simulink model "Model_kalmanTest"  (R2014b)
settings: Solver=ode3  StartTime=0.0  StopTime=T_max  FixedStep=h  RelTol=1e-3
values from neighbouring files (symbols this model uses):
  b = 0.1    [Input_LQR.m]    (also in TestKalman.m; TestSuper.m; TestVahidComparison.m; parameter.m)
  delta = cell(1,length(L_sup))    [TestSuper.m]
  g = 9.81    [Input_LQR.m]    (also in TestKalman.m; TestSuper.m; TestVahidComparison.m; parameter.m = 9.8)
  gamma = cell(1,length(L_sup))    [TestSuper.m]
  h = 0.01    [Input_LQR.m]    (also in TestKalman.m = 0.001; TestSuper.m = 0.001; TestVahidComparison.m = 0.001; parameter.m)
  H = [1 0 0 0 0 0 ... (first row only)    [Input_LQR.m]    (also in TestKalman.m; TestSuper.m; TestVahidComparison.m)
  K = lqr(A, B, Q, R)    [Input_LQR.m]    (also in TestKalman.m; TestSuper.m)
  k = 0.15    [Input_LQR.m]    (also in TestKalman.m; TestSuper.m; TestVahidComparison.m; parameter.m)
  L = 1.4    [Input_LQR.m]    (also in TestKalman.m; TestSuper.m = 1.025; TestVahidComparison.m)
  M = 1    [Input_LQR.m]    (also in TestKalman.m; TestSuper.m; TestVahidComparison.m; parameter.m)
  m = 3/4    (= 0.75)    [Input_LQR.m]    (also in TestKalman.m; TestSuper.m; TestVahidComparison.m; parameter.m)
  P_0 = diag([1,1,1,1,1,1])*0.00001    [Input_LQR.m]    (also in TestKalman.m = diag([1,1,1,1,100,100])*0.001; TestSuper.m = diag([1,1,1,1,100,100])*0.001)
  phi = cell(1,length(L_sup))    [TestSuper.m]
  Q_kalman = diag([(0), (0)])    [Input_LQR.m]    (also in TestKalman.m = diag([(10), (10e-4)]); TestSuper.m = diag([(10), (10e-4)]))
  R_kalman = diag([(10e-7), (10e-6)])    [Input_LQR.m]    (also in TestKalman.m = diag([(10e-7), (10e-7)]); TestSuper.m = diag([(10e-7), (10e-7)]))
  theta_0 = 0    [Input_LQR.m]    (also in TestKalman.m = 0.1; TestSuper.m = 0.1; TestVahidComparison.m = 0.1)
  theta_dot0 = 0    [Input_LQR.m]    (also in TestKalman.m; TestSuper.m; TestVahidComparison.m)
  X_0 = [0 0 0 0 0 0]'    [Input_LQR.m]    (also in TestKalman.m = [x_0 theta_0 x_dot0 theta_dot0 0 0]'; TestSuper.m = [x_0 theta_0 x_dot0 theta_dot0 0 0]')
  x_0 = 0    [Input_LQR.m]    (also in TestKalman.m; TestSuper.m; TestVahidComparison.m)
  x_dot0 = 0    [Input_LQR.m]    (also in TestKalman.m; TestSuper.m; TestVahidComparison.m)
  y_0 = [0 0]    [Input_LQR.m]    (also in TestKalman.m; TestSuper.m)
libraries: simulink x6
settings Model: Creator=Erik  LastModifiedBy=Erik
settings SolverCC: AlgebraicLoopSolver=LineSearch
settings OptimizationCC: UseDivisionForNetSlopeComputation=off  SimCompilerOptimization=off
settings DebuggingCC: FrameProcessingCompatibilityMsg=error
settings RTWCC: RTWCompilerOptimization=off
settings ConfigComp: CovMetricSettings=dw  CovHtmlReporting=on  CovSaveCumulativeToWorkspaceVar=on  CovSaveSingleToWorkspaceVar=on  CovModelRefEnable=Off  CovExternalEMLEnable=off  CovSFcnEnable=off

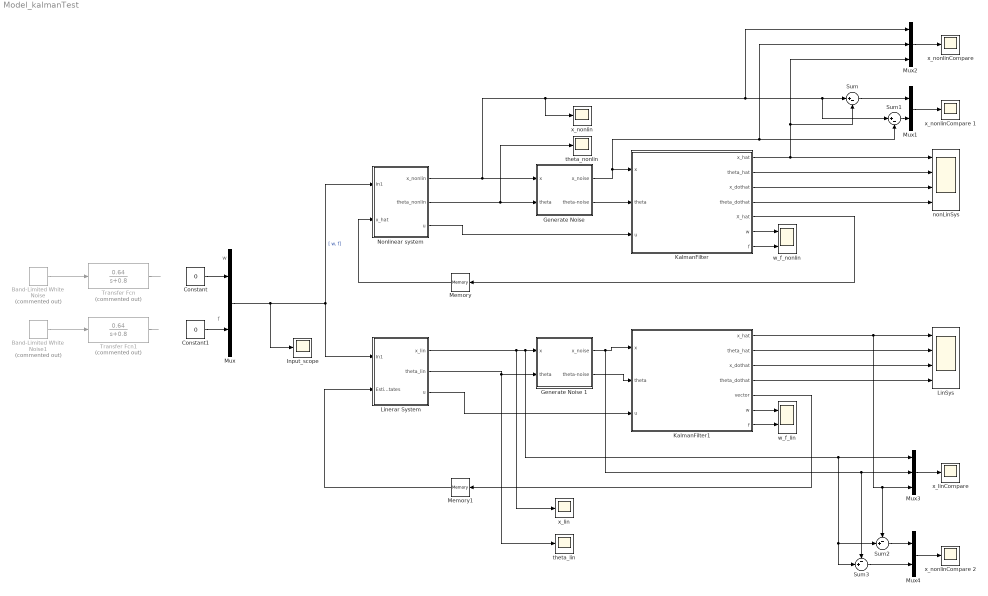
== system Model_kalmanTest ==
  note: f
  note: w
  Band-Limited White Noise : simulink/Sources/Band-Limited White Noise  Commented=on  Cov=Q_kalman(1,1)  Ts=h  seed=[23343]
  Band-Limited White Noise1 : simulink/Sources/Band-Limited White Noise  Commented=on  Cov=Q_kalman(2,2)  Ts=h  seed=[23344]
  Constant : Constant  Value=0
  Constant1 : Constant  Value=0
  "Generate Noise " : Subsystem
  Generate Noise 1 : Subsystem
  Input_scope : Scope
      settings: YMin=-4  YMax=3  SaveName=ScopeData4
  KalmanFilter : Subsystem
  KalmanFilter1 : Subsystem
  LinSys : Scope  NumInputPorts=4
      settings: YMin=-5~-5~-5~-5  YMax=5~5~5~5  SaveName=ScopeData9
  Linerar System : Subsystem
  Memory : Memory  X0=X_0
  Memory1 : Memory  X0=X_0
  Mux : Mux  Inputs=2
  Mux1 : Mux  Inputs=2
  Mux2 : Mux  Inputs=3
  Mux3 : Mux  Inputs=3
  Mux4 : Mux  Inputs=2
  "Nonlinear system " : Subsystem
  Sum : Sum  Inputs=|+-
  Sum1 : Sum  Inputs=|+-
  Sum2 : Sum  Inputs=-+|
  Sum3 : Sum  Inputs=-+|
  Transfer Fcn : TransferFcn  Commented=on  Numerator=[0.64]  Denominator=[1 0.8]
  Transfer Fcn1 : TransferFcn  Commented=on  Numerator=[0.64]  Denominator=[1 0.8]
  nonLinSys : Scope  NumInputPorts=4
      settings: YMin=-0.2~-0.1~-0.4~-0.5  YMax=1~0.2~1.2~0.1  SaveName=ScopeData8
  theta_lin : Scope
      settings: YMin=-228177358071237180000000000000000000000000000000000000000000000000000000000000000000000000000000000000000000000000000000000000000000000000000000000000000000000000000000000000000000000000000000000000000000000000000000000000000000000000000000000000000000000000000000000000000000000000000000000000000000000000.00000  YMax=25353039785693015000000000000000000000000000000000000000000000000000000000000000000000000000000000000000000000000000000000000000000000000000000000000000000000000000000000000000000000000000000000000000000000000000000000000000000000000000000000000000000000000000000000000000000000000000000000000000000000000.00000  SaveName=ScopeData2
  "theta_nonlin " : Scope
      settings: YMin=-0.04693  YMax=0.15685  SaveName=ScopeData3
  w_f_lin : Scope  NumInputPorts=2
      settings: ShowLegends=on  YMin=-5000~-5  YMax=2000~5  SaveName=ScopeData10
  w_f_nonlin : Scope  NumInputPorts=2
      settings: ShowLegends=on  YMin=-5000~-5  YMax=2000~5  SaveName=ScopeData12
  x_lin : Scope
      settings: YMin=-0.5  YMax=0.5
  x_linCompare : Scope
      settings: ShowLegends=on  YMin=-5000  YMax=2000  SaveName=ScopeData6
  x_nonlin : Scope
      settings: TimeRange=100  YMin=-4  YMax=3
  "x_nonlinCompare " : Scope
      settings: ShowLegends=on  YMin=-1.5  YMax=2.5  SaveName=ScopeData5
  x_nonlinCompare 1 : Scope
      settings: ShowLegends=on  YMin=-0.04  YMax=0.04  SaveName=ScopeData11
  x_nonlinCompare 2 : Scope
      settings: ShowLegends=on  YMin=-0.015  YMax=0.015  SaveName=ScopeData7
  wires:
  Mux/1 -> Linerar System/1(In1), "Nonlinear system "/1(In1), Input_scope/1  "[ w, f]"
  "Nonlinear system "/1(x_nonlin) -> x_nonlin/1, Sum1/1, Sum/1, Mux2/1, "Generate Noise "/1(x)
  "Nonlinear system "/2(theta_nonlin) -> "theta_nonlin "/1, "Generate Noise "/2(theta)
  Linerar System/2(theta_lin) -> theta_lin/1, Generate Noise 1/2(theta)
  KalmanFilter/1(x_hat) -> nonLinSys/1, Mux2/3, Sum/2
  KalmanFilter/2(theta_hat) -> nonLinSys/2
  KalmanFilter/4(theta_dothat) -> nonLinSys/4
  KalmanFilter1/5(vector) -> Memory1/1
  KalmanFilter/3(x_dothat) -> nonLinSys/3
  "Nonlinear system "/3(u) -> KalmanFilter/3("u ")
  Memory/1 -> "Nonlinear system "/2(x_hat)
  Band-Limited White Noise/1 -> Transfer Fcn/1
  Band-Limited White Noise1/1 -> Transfer Fcn1/1
  Transfer Fcn1/1 -> ?
  Transfer Fcn/1 -> ?
  "Generate Noise "/1(x_noise) -> KalmanFilter/1(x), Mux2/2, Sum1/2
  "Generate Noise "/2(theta-noise) -> KalmanFilter/2(theta)
  Generate Noise 1/2(theta-noise) -> KalmanFilter1/2(theta)
  Linerar System/3(u) -> KalmanFilter1/3("u ")
  Mux2/1 -> "x_nonlinCompare "/1
  Linerar System/1(x_lin) -> x_lin/1, Mux3/1, Sum2/2, Sum3/2, Generate Noise 1/1(x)
  KalmanFilter1/1(x_hat) -> LinSys/1, Mux3/3, Sum2/1
  Generate Noise 1/1(x_noise) -> Mux3/2, Sum3/1, KalmanFilter1/1(x)
  Mux3/1 -> x_linCompare/1
  Memory1/1 -> Linerar System/2(Estimated states)
  KalmanFilter/5(X_hat) -> Memory/1
  Sum/1 -> Mux1/1
  Mux1/1 -> x_nonlinCompare 1/1
  Sum1/1 -> Mux1/2
  Sum2/1 -> Mux4/1
  Mux4/1 -> x_nonlinCompare 2/1
  Sum3/1 -> Mux4/2
  KalmanFilter1/2(theta_hat) -> LinSys/2
  KalmanFilter1/3(x_dothat) -> LinSys/3
  KalmanFilter1/4(theta_dothat) -> LinSys/4
  KalmanFilter/6(w) -> w_f_nonlin/1
  KalmanFilter/7(f) -> w_f_nonlin/2
  KalmanFilter1/6(w) -> w_f_lin/1
  KalmanFilter1/7(f) -> w_f_lin/2
  Constant1/1 -> Mux/2
  Constant/1 -> Mux/1

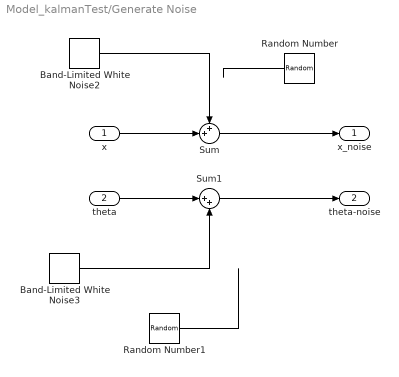
== system Model_kalmanTest/Generate Noise  ==
  x : Inport
  theta : Inport  Port=2
  Band-Limited White Noise2 : simulink/Sources/Band-Limited White Noise  Cov=R_kalman(1,1)  Ts=h  seed=[23342]
  Band-Limited White Noise3 : simulink/Sources/Band-Limited White Noise  Cov=R_kalman(2,2)  Ts=h  seed=[23341]
  Random Number : RandomNumber  Variance=R_kalman(1,1)  SampleTime=h
  Random Number1 : RandomNumber  Variance=R_kalman(2,2)  SampleTime=h
  Sum : Sum  Inputs=++|
  Sum1 : Sum  Inputs=|++
  x_noise : Outport
  theta-noise : Outport  Port=2
  wires:
  Sum/1 -> x_noise/1
  x/1 -> Sum/2
  Band-Limited White Noise2/1 -> Sum/1
  theta/1 -> Sum1/1
  Sum1/1 -> theta-noise/1
  Band-Limited White Noise3/1 -> Sum1/2
  Random Number/1 -> ?
  Random Number1/1 -> ?

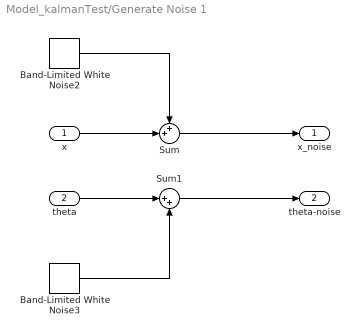
== system Model_kalmanTest/Generate Noise 1 ==
  x : Inport
  theta : Inport  Port=2
  Band-Limited White Noise2 : simulink/Sources/Band-Limited White Noise  Cov=R_kalman(1,1)  Ts=h  seed=[23342]
  Band-Limited White Noise3 : simulink/Sources/Band-Limited White Noise  Cov=R_kalman(2,2)  Ts=h  seed=[23341]
  Sum : Sum  Inputs=++|
  Sum1 : Sum  Inputs=|++
  x_noise : Outport
  theta-noise : Outport  Port=2
  wires:
  Sum/1 -> x_noise/1
  x/1 -> Sum/2
  Band-Limited White Noise2/1 -> Sum/1
  theta/1 -> Sum1/1
  Sum1/1 -> theta-noise/1
  Band-Limited White Noise3/1 -> Sum1/2

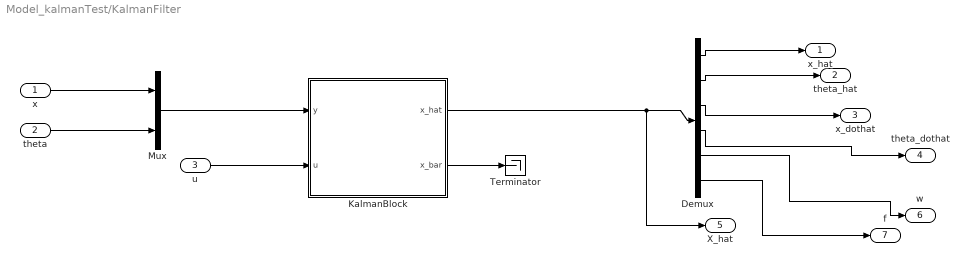
== system Model_kalmanTest/KalmanFilter ==
  x : Inport
  theta : Inport  Port=2
  "u " : Inport  Port=3
  Demux : Demux  Outputs=6
  KalmanBlock : Subsystem
  Mux : Mux  Inputs=2
  Terminator : Terminator
  x_hat : Outport
  theta_hat : Outport  Port=2
  x_dothat : Outport  Port=3
  theta_dothat : Outport  Port=4
  X_hat : Outport  Port=5
  w : Outport  Port=6
  f : Outport  Port=7
  wires:
  Mux/1 -> KalmanBlock/1("y ")
  "u "/1 -> KalmanBlock/2("u ")
  x/1 -> Mux/1
  theta/1 -> Mux/2
  KalmanBlock/1(x_hat) -> X_hat/1, Demux/1
  Demux/1 -> x_hat/1
  Demux/2 -> theta_hat/1
  Demux/3 -> x_dothat/1
  Demux/4 -> theta_dothat/1
  KalmanBlock/2(x_bar) -> Terminator/1
  Demux/5 -> w/1
  Demux/6 -> f/1

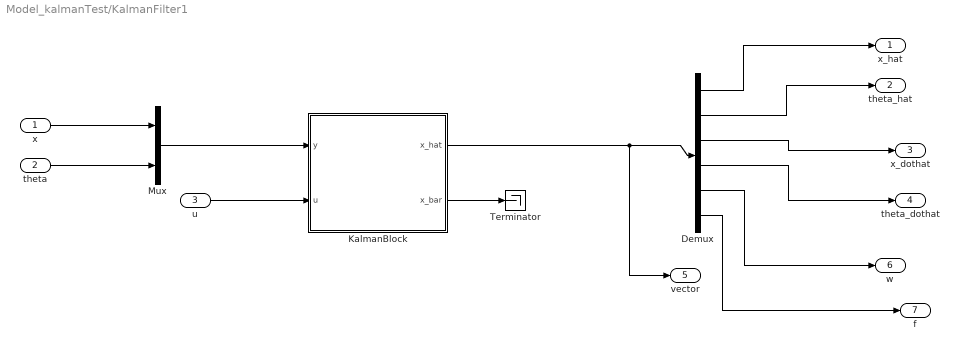
== system Model_kalmanTest/KalmanFilter1 ==
  x : Inport
  theta : Inport  Port=2
  "u " : Inport  Port=3
  Demux : Demux  Outputs=6
  KalmanBlock : Subsystem
  Mux : Mux  Inputs=2
  Terminator : Terminator
  x_hat : Outport
  theta_hat : Outport  Port=2
  x_dothat : Outport  Port=3
  theta_dothat : Outport  Port=4
  vector : Outport  Port=5
  w : Outport  Port=6
  f : Outport  Port=7
  wires:
  Mux/1 -> KalmanBlock/1("y ")
  "u "/1 -> KalmanBlock/2("u ")
  x/1 -> Mux/1
  theta/1 -> Mux/2
  KalmanBlock/1(x_hat) -> vector/1, Demux/1
  Demux/1 -> x_hat/1
  Demux/2 -> theta_hat/1
  Demux/3 -> x_dothat/1
  Demux/4 -> theta_dothat/1
  KalmanBlock/2(x_bar) -> Terminator/1
  Demux/5 -> w/1
  Demux/6 -> f/1

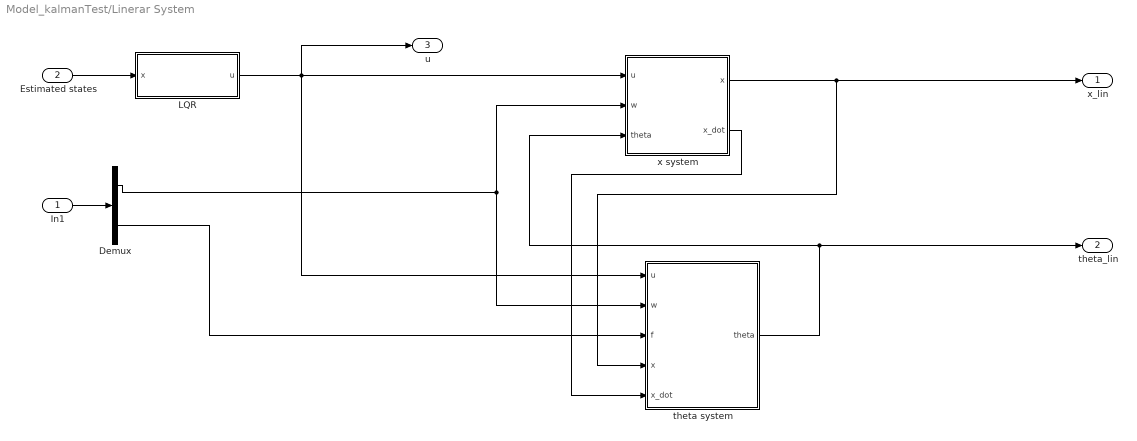
== system Model_kalmanTest/Linerar System ==
  In1 : Inport
  Estimated states : Inport  Port=2
  Demux : Demux  Outputs=2
  LQR : Subsystem
  "theta system " : Subsystem
  x system : Subsystem
  x_lin : Outport
  theta_lin : Outport  Port=2
  u : Outport  Port=3
  wires:
  x system/1(x) -> "theta system "/4(x), x_lin/1
  Demux/1 -> "theta system "/2(w), x system/2(w)
  "theta system "/1(theta) -> theta_lin/1, x system/3(theta)
  Demux/2 -> "theta system "/3(f)
  x system/2(x_dot) -> "theta system "/5(x_dot)
  In1/1 -> Demux/1
  LQR/1(u) -> u/1, "theta system "/1("u "), x system/1("u ")
  Estimated states/1 -> LQR/1(x)

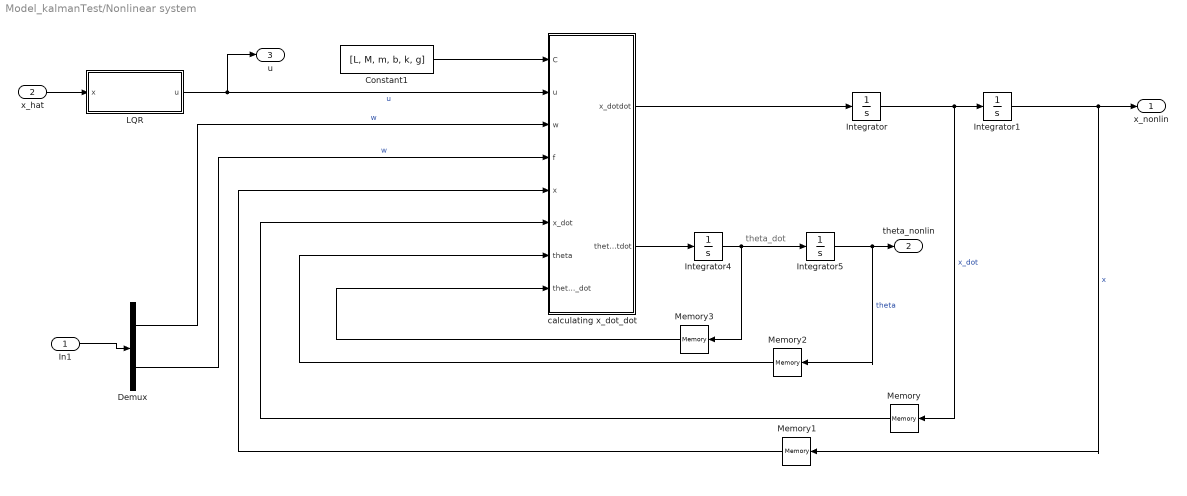
== system Model_kalmanTest/Nonlinear system  ==
  note: theta_dot
  In1 : Inport
  x_hat : Inport  Port=2
  Constant1 : Constant  Value=[L, M, m, b, k, g]  SampleTime=0.01
  Demux : Demux  Outputs=2
  Integrator : Integrator  InitialCondition=x_dot0
  Integrator1 : Integrator  InitialCondition=x_0
  Integrator4 : Integrator  InitialCondition=theta_dot0
  Integrator5 : Integrator  InitialCondition=theta_0
  LQR : Subsystem
  Memory : Memory  X0=x_dot0
  Memory1 : Memory  X0=x_0
  Memory2 : Memory  X0=theta_0
  Memory3 : Memory  X0=theta_dot0
  calculating x_dot_dot : MATLAB Function  TreatAsAtomicUnit=on
  x_nonlin : Outport
  theta_nonlin : Outport  Port=2
  u : Outport  Port=3
  wires:
  In1/1 -> Demux/1
  LQR/1(u) -> u/1, calculating x_dot_dot/2(u)  "u"
  Demux/1 -> calculating x_dot_dot/3(w)  "w"
  calculating x_dot_dot/1(x_dotdot) -> Integrator/1
  Integrator/1 -> Memory/1, Integrator1/1  "x_dot"
  Integrator1/1 -> Memory1/1, x_nonlin/1  "x"
  Constant1/1 -> calculating x_dot_dot/1(C)
  calculating x_dot_dot/2(theta_dotdot) -> Integrator4/1
  Integrator4/1 -> Memory3/1, Integrator5/1
  Integrator5/1 -> Memory2/1, theta_nonlin/1  "theta"
  Memory1/1 -> calculating x_dot_dot/5(x)
  Memory/1 -> calculating x_dot_dot/6(x_dot)
  Memory2/1 -> calculating x_dot_dot/7(theta)
  Memory3/1 -> calculating x_dot_dot/8(theta_dot)
  x_hat/1 -> LQR/1(x)
  Demux/2 -> calculating x_dot_dot/4(f)  "w"

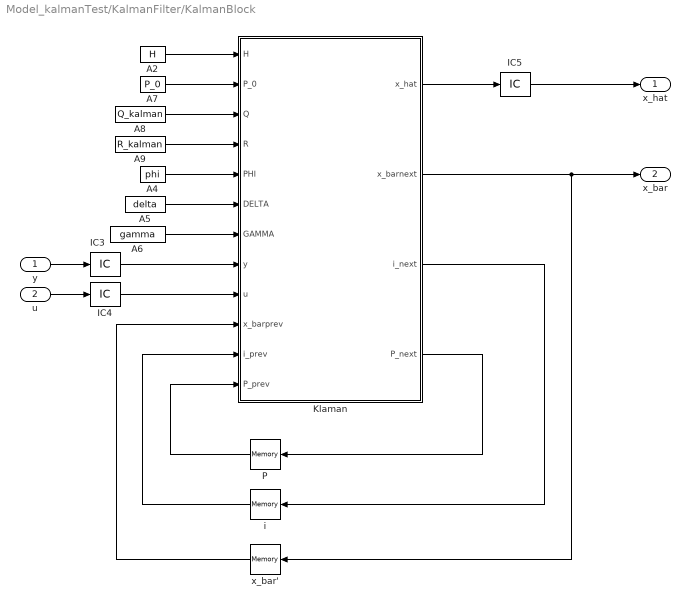
== system Model_kalmanTest/KalmanFilter/KalmanBlock ==
  "y " : Inport
  "u " : Inport  Port=2
  A2 : Constant  Value=H
  A4 : Constant  Value=phi
  A5 : Constant  Value=delta
  A6 : Constant  Value=gamma
  A7 : Constant  Value=P_0
  A8 : Constant  Value=Q_kalman
  A9 : Constant  Value=R_kalman
  IC3 : InitialCondition  Value=y_0
  IC4 : InitialCondition  Value=0
  IC5 : InitialCondition  Value=X_0
  Klaman : MATLAB Function  TreatAsAtomicUnit=on
  P : Memory  X0=P_0
  "i " : Memory
  x_bar' : Memory  X0=X_0
  x_hat : Outport
  x_bar : Outport  Port=2
  wires:
  A8/1 -> Klaman/3(Q)
  A6/1 -> Klaman/7(GAMMA)
  A4/1 -> Klaman/5(PHI)
  Klaman/2(x_barnext) -> x_bar'/1, x_bar/1
  Klaman/3(i_next) -> "i "/1
  Klaman/1(x_hat) -> IC5/1
  Klaman/4(P_next) -> P/1
  A2/1 -> Klaman/1(H)
  A5/1 -> Klaman/6(DELTA)
  IC4/1 -> Klaman/9(u)
  A7/1 -> Klaman/2(P_0)
  "u "/1 -> IC4/1
  A9/1 -> Klaman/4(R)
  "y "/1 -> IC3/1
  IC5/1 -> x_hat/1
  IC3/1 -> Klaman/8(y)
  "i "/1 -> Klaman/11(i_prev)
  P/1 -> Klaman/12(P_prev)
  x_bar'/1 -> Klaman/10(x_barprev)

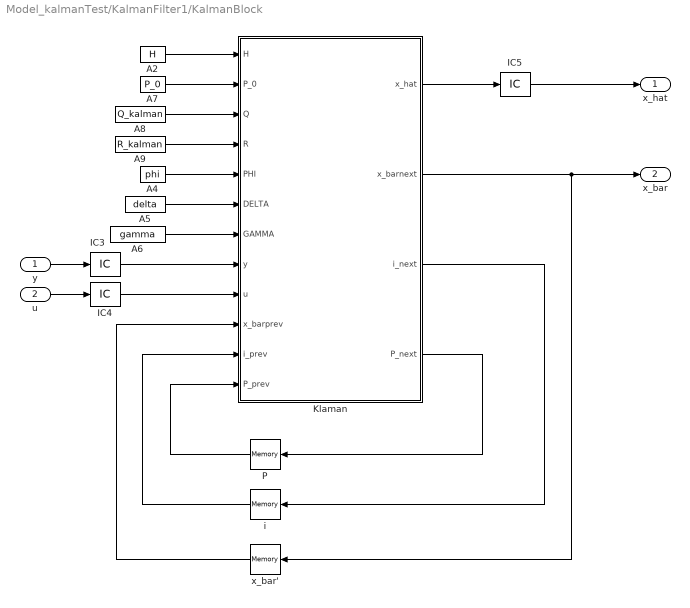
== system Model_kalmanTest/KalmanFilter1/KalmanBlock ==
  "y " : Inport
  "u " : Inport  Port=2
  A2 : Constant  Value=H
  A4 : Constant  Value=phi
  A5 : Constant  Value=delta
  A6 : Constant  Value=gamma
  A7 : Constant  Value=P_0
  A8 : Constant  Value=Q_kalman
  A9 : Constant  Value=R_kalman
  IC3 : InitialCondition  Value=y_0
  IC4 : InitialCondition  Value=0
  IC5 : InitialCondition  Value=X_0
  Klaman : MATLAB Function  TreatAsAtomicUnit=on
  P : Memory  X0=P_0
  "i " : Memory
  x_bar' : Memory  X0=X_0
  x_hat : Outport
  x_bar : Outport  Port=2
  wires:
  A8/1 -> Klaman/3(Q)
  A6/1 -> Klaman/7(GAMMA)
  A4/1 -> Klaman/5(PHI)
  Klaman/2(x_barnext) -> x_bar'/1, x_bar/1
  Klaman/3(i_next) -> "i "/1
  Klaman/1(x_hat) -> IC5/1
  Klaman/4(P_next) -> P/1
  A2/1 -> Klaman/1(H)
  A5/1 -> Klaman/6(DELTA)
  IC4/1 -> Klaman/9(u)
  A7/1 -> Klaman/2(P_0)
  "u "/1 -> IC4/1
  A9/1 -> Klaman/4(R)
  "y "/1 -> IC3/1
  IC5/1 -> x_hat/1
  IC3/1 -> Klaman/8(y)
  "i "/1 -> Klaman/11(i_prev)
  P/1 -> Klaman/12(P_prev)
  x_bar'/1 -> Klaman/10(x_barprev)

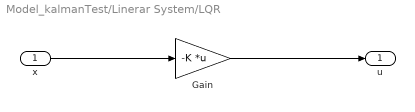
== system Model_kalmanTest/Linerar System/LQR ==
  x : Inport
  Gain : Gain  Gain=-K  Multiplication=Matrix(K*u)
  u : Outport
  wires:
  Gain/1 -> u/1
  x/1 -> Gain/1

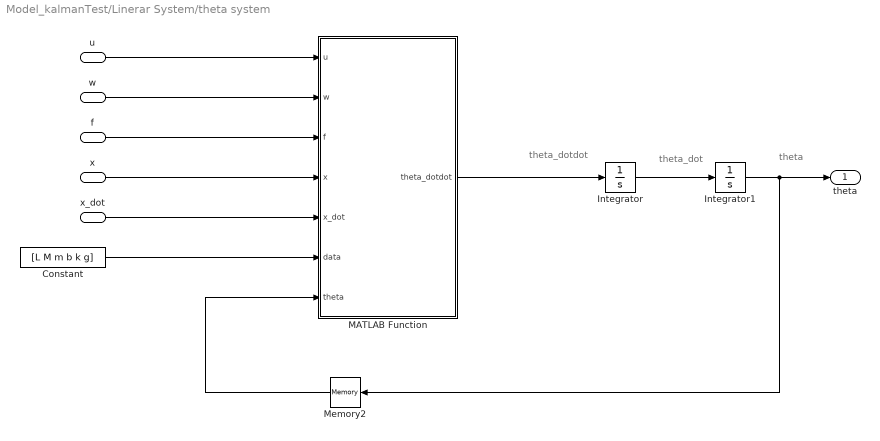
== system Model_kalmanTest/Linerar System/theta system  ==
  note: theta
  note: theta_dotdot
  note: theta_dot
  "u " : Inport
  w : Inport  Port=2
  f : Inport  Port=3
  x : Inport  Port=4
  x_dot : Inport  Port=5
  Constant : Constant  Value=[L M m b k g]  VectorParams1D=off  SampleTime=0.01
  Integrator : Integrator  InitialCondition=theta_dot0
  Integrator1 : Integrator  InitialCondition=theta_0
  MATLAB Function : MATLAB Function  TreatAsAtomicUnit=on
  Memory2 : Memory  X0=theta_0
  theta : Outport
  wires:
  MATLAB Function/1(theta_dotdot) -> Integrator/1
  "u "/1 -> MATLAB Function/1(u)
  w/1 -> MATLAB Function/2(w)
  x/1 -> MATLAB Function/4(x)
  Integrator1/1 -> Memory2/1, theta/1
  Constant/1 -> MATLAB Function/6(data)
  f/1 -> MATLAB Function/3(f)
  x_dot/1 -> MATLAB Function/5(x_dot)
  Memory2/1 -> MATLAB Function/7(theta)
  Integrator/1 -> Integrator1/1

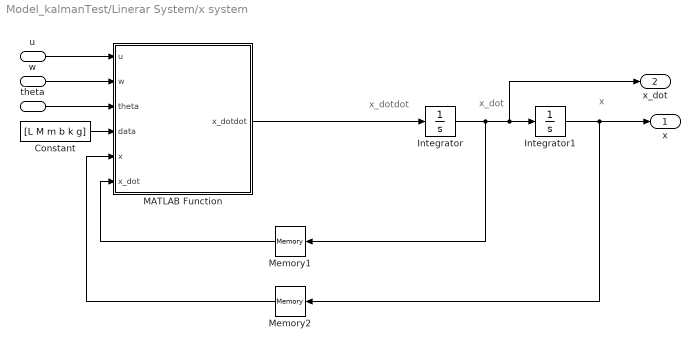
== system Model_kalmanTest/Linerar System/x system ==
  note: x
  note: x_dotdot
  note: x_dot
  "u " : Inport
  w : Inport  Port=2
  theta : Inport  Port=3
  Constant : Constant  Value=[L M m b k g]  VectorParams1D=off  SampleTime=0.01
  Integrator : Integrator  InitialCondition=x_dot0
  Integrator1 : Integrator  InitialCondition=x_0
  MATLAB Function : MATLAB Function  TreatAsAtomicUnit=on
  Memory1 : Memory  X0=x_dot0
  Memory2 : Memory  X0=x_0
  x : Outport
  x_dot : Outport  Port=2
  wires:
  Memory1/1 -> MATLAB Function/6(x_dot)
  "u "/1 -> MATLAB Function/1(u)
  w/1 -> MATLAB Function/2(w)
  theta/1 -> MATLAB Function/3(theta)
  Integrator1/1 -> Memory2/1, x/1
  Memory2/1 -> MATLAB Function/5(x)
  Constant/1 -> MATLAB Function/4(data)
  Integrator/1 -> Integrator1/1, x_dot/1, Memory1/1
  MATLAB Function/1(x_dotdot) -> Integrator/1

== system Model_kalmanTest/Nonlinear system /LQR ==
  x : Inport
  Gain : Gain  Gain=-K  Multiplication=Matrix(K*u)
  u : Outport
  wires:
  Gain/1 -> u/1
  x/1 -> Gain/1

== matlab function Model_kalmanTest/Linerar System/x system/MATLAB Function ==
  data: u input; w input; theta input; data input; x_dotdot output; x input; x_dot input
function x_dotdot  = fcn(u, w, theta, data, x, x_dot)
L = data(1);
M = data(2);
m = data(3);
b = data(4);
k = data(5);
g = data(6);

% theta = theta * 180 / pi;

x_dotdot=(u - w - m * g * theta - b * x_dot - k * x) / M;


end

== matlab function Model_kalmanTest/KalmanFilter/KalmanBlock/Klaman ==
  data: H input; P_0 input; Q input; R input; PHI input; DELTA input; GAMMA input; y input; u input; x_barprev input; i_prev input; P_prev input; x_hat output; x_barnext output; i_next output; P_next output
function [x_hat,x_barnext,i_next,P_next] = KalmanFilter(H,P_0,Q,R,PHI,DELTA,GAMMA,y,u,x_barprev,i_prev,P_prev)
[a,b]=size(P_0);
I=eye(a);
if i_prev ==0
    x_barnext=x_barprev;
    x_hat=x_barprev;
    P_next=P_0;
else
    %[kest,L,P,M,Z]=kalmd(sys,Q_kalman,R_kalman,h)
    K=P_prev*(H')*inv(H*P_prev*(H')+R);
    x_hat=x_barprev+K*(y-H*x_barprev);
    P_hat=(I-K*H)*P_prev*(I-K*H)'+K*R*K';
    
    x_barnext=PHI*x_hat+DELTA*u;
    P_next=PHI*P_hat*PHI'+GAMMA*Q*GAMMA';
end

i_next=i_prev+1;
end

== matlab function Model_kalmanTest/Linerar System/theta system /MATLAB Function ==
  data: u input; w input; f input; x input; x_dot input; data input; theta input; theta_dotdot output
function theta_dotdot  = fcn(u, w, f, x, x_dot, data, theta)
L = data(1);
M = data(2);
m = data(3);
b = data(4);
k = data(5);
g = data(6);

% theta = theta * 180 / pi;

theta_dotdot=(-u + w + (m + M) * g * theta - (M / m) * f + b * x_dot + k * x)/(L * M);

end

== matlab function Model_kalmanTest/Nonlinear system /calculating x_dot_dot ==
  data: C input; u input; x_dotdot output; w input; f input; x input; x_dot input; theta input; theta_dot input; theta_dotdot output
function [x_dotdot, theta_dotdot]= fcn(C,u, w, f, x, x_dot, theta, theta_dot)
%extracting the know parameters from vector C
L = C(1); 
M= C(2); 
m=C(3); 
b = C(4); 
k = C(5); 
g = C(6);

%calculating x_dot_dot
 x_dotdot = (u - f - w + f*cos(theta)^2 ...
            + m*L*theta_dot^2*sin(theta) ...
            -m*g*sin(theta)*cos(theta)...
            -b*x_dot -k*x )/(M + m*sin(theta)^2); 

%calculating theta_dot_dot
 theta_dotdot = (-u*cos(theta)+w*cos(theta)...
                   -M*L*theta_dot^2*sin(theta)*cos(theta)...
                    +(m+M)*g*sin(theta)-(M/m)*f*cos(theta)...
                    +b*x_dot*cos(theta)...
                    + k*x*cos(theta))/(L*(M+m*sin(theta)^2));

== matlab function Model_kalmanTest/KalmanFilter1/KalmanBlock/Klaman ==
  data: H input; P_0 input; Q input; R input; PHI input; DELTA input; GAMMA input; y input; u input; x_barprev input; i_prev input; P_prev input; x_hat output; x_barnext output; i_next output; P_next output
function [x_hat, x_barnext, i_next, P_next] = KalmanFilter(H, P_0, Q, R, PHI, DELTA, GAMMA, y, u, x_barprev, i_prev, P_prev)
I = eye(6);
if i_prev == 0
    x_barnext = x_barprev;
    x_hat = x_barprev;
    P_next = P_0;
else
    K = P_prev * (H') * inv(H * P_prev * (H') + R);
    x_hat = x_barprev + K * (y - H * x_barprev);
    P_hat = (I - K * H) * P_prev * (I - K * H)' + K * R * K';
    
    x_barnext = PHI * x_hat + DELTA * u;
    P_next = PHI * P_hat * PHI' + GAMMA * Q * GAMMA';
end

i_next=i_prev+1;
end
